simulink model "motor_test"  (R2025b)
settings: Solver=VariableStepAuto  StartTime=0.0  StopTime=10.0  RelTol=1e-3
model workspace (MAT data in the model file):
  J = 1e-05
  Km = 0.0023682432808
  L = 1.4545234036e-06
  R = 4.57005751872
  Vn = 24
  bv = 0.0001
libraries: simulink x4, subsystems x1
settings Model: Creator=karadeli  LastModifiedBy=karadeli

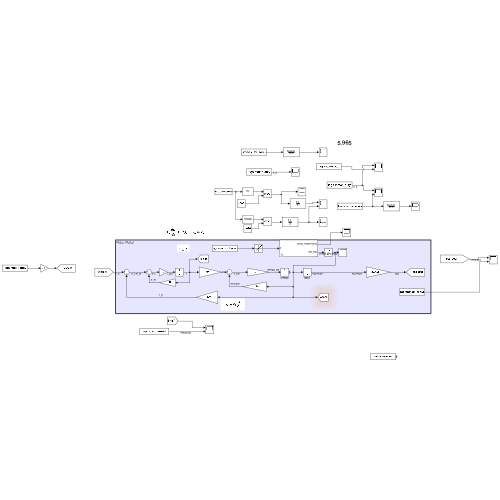
[thumbnail: Simulink's stored preview of the top-level diagram]
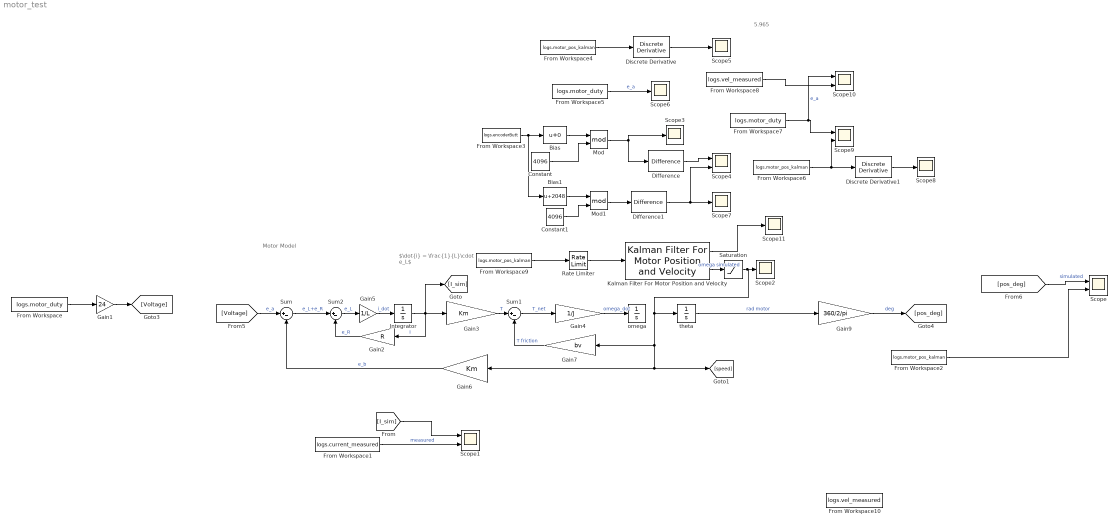
== system motor_test ==
  note: 5.965
  note: $\dot{i} = \frac{1}{L}\cdot e_L$
  note: Motor Model
  Bias : Bias  SaturateOnIntegerOverflow=off
  Bias1 : Bias  Bias=2048  SaturateOnIntegerOverflow=off
  Constant : Constant  Value=4096
  Constant1 : Constant  Value=4096
  Difference : simulink/Discrete/Difference  ICPrevInput=0.0  OutMin=[]  OutMax=[]  OutDataType=fixdt(1, 16)  OutScaling=2^-10  DoSatur=off
  Difference1 : simulink/Discrete/Difference  ICPrevInput=0.0  OutMin=[]  OutMax=[]  OutDataType=fixdt(1, 16)  OutScaling=2^-10  DoSatur=off
  Discrete Derivative : simulink/Discrete/Discrete Derivative  gainval=1.0  ICPrevScaledInput=0.0  OutMin=[]  OutMax=[]  OutDataType=fixdt(1, 16)  OutScaling=2^-10  DoSatur=off
  Discrete Derivative1 : simulink/Discrete/Discrete Derivative  gainval=1.0  ICPrevScaledInput=0.0  OutMin=[]  OutMax=[]  OutDataType=fixdt(1, 16)  OutScaling=2^-10  DoSatur=off
  From Workspace : FromWorkspace  VariableName=logs.motor_duty  SampleTime=1e-3  Interpolate=off  OutputAfterFinalValue=Holding final value
  From Workspace1 : FromWorkspace  VariableName=logs.current_measured  SampleTime=1e-3  Interpolate=off  OutputAfterFinalValue=Holding final value
  From Workspace10 : FromWorkspace  VariableName=logs.vel_measured
  From Workspace{2,4,6,9} (4 alike) : FromWorkspace  VariableName=logs.motor_pos_kalman
  From Workspace3 : FromWorkspace  VariableName=logs.encoderButt  SampleTime=1e-3  Interpolate=off  OutputAfterFinalValue=Holding final value
  From Workspace5 : FromWorkspace  VariableName=logs.motor_duty  SampleTime=1e-3  Interpolate=off  OutputAfterFinalValue=Holding final value
  From Workspace7 : FromWorkspace  VariableName=logs.motor_duty  SampleTime=1e-3  Interpolate=off  OutputAfterFinalValue=Holding final value
  From Workspace8 : FromWorkspace  VariableName=logs.vel_measured
  Gain1 : Gain  Gain=24
  Gain2 : Gain  Gain=R
  Gain3 : Gain  Gain=Km
  Gain4 : Gain  Gain=1/J
  Gain5 : Gain  Gain=1/L
  Gain6 : Gain  Gain=Km
  Gain7 : Gain  Gain=bv
  Gain9 : Gain  Gain=360/2/pi
  Integrator : Integrator
  Kalman Filter For Motor Position and Velocity : subsystems/Kalman Filter For Motor Position and Velocity  Ts=1e-3
  Mod : Math  Operator=mod
  Mod1 : Math  Operator=mod
  Rate Limiter : RateLimiter  RisingSlewLimit=6e3/60*360  FallingSlewLimit=-6e3*6  SampleTimeMode=inherited
  Saturation : Saturate  UpperLimit=1500  LowerLimit=-1500
  Scope{,1,4,9..10} (5 alike) : Scope  NumInputPorts=2
      Scope settings: ActiveDisplayYMinimum=-1  ActiveDisplayYMaximum=1
      Scope1 settings: ActiveDisplayYMinimum=-10.483620778973091  ActiveDisplayYMaximum=9.5195730913949248
      Scope10 settings: ActiveDisplayYMinimum=-0.74999987334012985  ActiveDisplayYMaximum=0.74999981373548508  DataLoggingVariableName=ScopeData10
      Scope4 settings: ActiveDisplayYMinimum=-5119.89013671875  ActiveDisplayYMaximum=5119.89013671875  DataLoggingVariableName=ScopeData4
      Scope9 settings: ActiveDisplayYMinimum=-0.75000002980232239  ActiveDisplayYMaximum=0.75000002980232239  DataLoggingVariableName=ScopeData9
  Scope{2..3,5..8,11} (7 alike) : Scope
      Scope11 settings: ActiveDisplayYMinimum=-1  ActiveDisplayYMaximum=1  DataLoggingVariableName=ScopeData11
      Scope2 settings: ActiveDisplayYMinimum=-1875  ActiveDisplayYMaximum=1875  DataLoggingVariableName=ScopeData2
      Scope3 settings: ActiveDisplayYMinimum=-133.3405172413793  ActiveDisplayYMaximum=4972.90948275862  DataLoggingVariableName=ScopeData3
      Scope5 settings: ActiveDisplayYMinimum=-8282.02910271316  ActiveDisplayYMaximum=8518.3095255259541  DataLoggingVariableName=ScopeData5
      Scope6 settings: ActiveDisplayYMinimum=-1  ActiveDisplayYMaximum=1  DataLoggingVariableName=ScopeData6
      Scope7 settings: ActiveDisplayYMinimum=-5089.117431640625  ActiveDisplayYMaximum=5090.787353515625  DataLoggingVariableName=ScopeData7
      Scope8 settings: ActiveDisplayYMinimum=2744.1825411211489  ActiveDisplayYMaximum=3003.588804274601  DataLoggingVariableName=ScopeData8
  Sum : Sum  Inputs=|+-
  Sum1 : Sum  Inputs=|+-
  Sum2 : Sum  Inputs=|+-
  omega : Integrator
  theta : Integrator  ZeroCross=off
  wires:
  From Workspace1/1 -> Scope1/2  "measured"
  Gain1/1 -> [Voltage]
  Sum2/1 -> Gain5/1  "e_L"
  Kalman Filter For Motor Position and Velocity/2 -> Saturation/1  "omega simulated"
  Gain9/1 -> [pos_deg]  "deg"
  [Voltage] -> Sum/1  "e_a"
  Gain4/1 -> omega/1  "omega_dot"
  Sum1/1 -> Gain4/1  "T_net"
  Sum/1 -> Sum2/1  "e_L+e_R"
  Gain7/1 -> Sum1/2  "T friction"
  From Workspace/1 -> Gain1/1
  Gain6/1 -> Sum/2  "e_b"
  Gain3/1 -> Sum1/1  "T"
  theta/1 -> Gain9/1  "rad motor"
  [pos_deg] -> Scope/1  "simulated"
  Integrator/1 -> Gain2/1, [I_sim], Gain3/1  "I"
  Gain2/1 -> Sum2/2  "e_R"
  Gain5/1 -> Integrator/1  "i_dot"
  From Workspace2/1 -> Scope/2
  [I_sim] -> Scope1/1
  From Workspace3/1 -> Bias1/1, Bias/1
  Difference/1 -> Scope4/1
  Mod/1 -> Scope3/1, Difference/1
  Bias/1 -> Mod/1
  Constant/1 -> Mod/2
  From Workspace4/1 -> Discrete Derivative/1
  Discrete Derivative/1 -> Scope5/1
  From Workspace5/1 -> Scope6/1  "e_a"
  Bias1/1 -> Mod1/1
  Constant1/1 -> Mod1/2
  Mod1/1 -> Difference1/1
  Difference1/1 -> Scope4/2, Scope7/1
  From Workspace6/1 -> Scope9/2, Discrete Derivative1/1
  Discrete Derivative1/1 -> Scope8/1
  From Workspace7/1 -> Scope10/1, Scope9/1  "e_a"
  From Workspace8/1 -> Scope10/2
  From Workspace9/1 -> Rate Limiter/1
  Kalman Filter For Motor Position and Velocity/1 -> Scope11/1
  Saturation/1 -> Scope2/1, [speed], Gain6/1, Gain7/1, theta/1
  Rate Limiter/1 -> Kalman Filter For Motor Position and Velocity/1
